simulink model "sfcndemo_sfun_udt"  (Simulink 6.0)
settings: Solver=ode1  StartTime=0.0  StopTime=10.0  FixedStep=0.05  RelTol=1e-3
settings Model: Creator=The MathWorks Inc.  LastModifiedBy=batserve  ExtModeAutoUpdateStatusClock=off
settings SolverCC: ZeroCrossControl=DisableAll
settings DataIOCC: SaveOutput=off  SaveTime=off
settings OptimizationCC: BlockReduction=off  BooleanDataType=off  InlineInvariantSignals=off
settings DebuggingCC: CheckExecutionContextPreStartOutputMsg=on  CheckExecutionContextRuntimeOutputMsg=on  SolverPrmCheckMsg=none
settings HardwareCC: TargetUnknown=on
settings RTWCC: RetainRTWFile=on

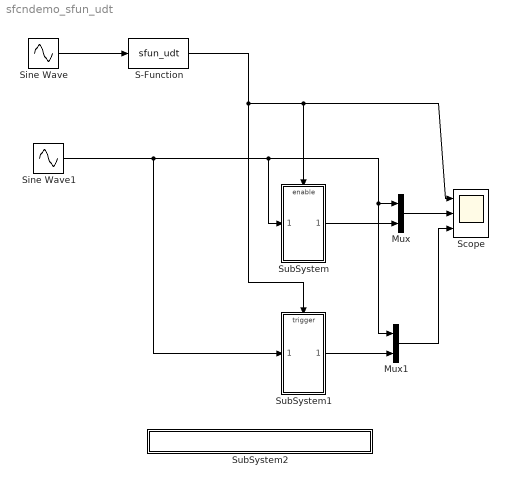
== system sfcndemo_sfun_udt ==
  Mux : Mux  Inputs=2
  Mux1 : Mux  Inputs=2
  S-Function : S-Function  FunctionName=sfun_udt
  Scope : Scope  NumInputPorts=3
      settings: YMin=-5~-5~-5  YMax=5~5~5
  Sine Wave : Sin  Amplitude=4.5  Frequency=1.5  SampleTime=0.05
  Sine Wave1 : Sin  Amplitude=4  SampleTime=0.05
  SubSystem : Subsystem  TreatAsAtomicUnit=on  PropExecContextAcrossSSBoundary=on
  SubSystem1 : Subsystem  TreatAsAtomicUnit=on  PropExecContextAcrossSSBoundary=on
  SubSystem2 : Subsystem  PropExecContextAcrossSSBoundary=on
      settings: OpenFcn=edit(fullfile(matlabroot,'simulink','src','sfun_udt.c'))
      mask Display: disp('matlabroot\simulink\src\sfun_udt.c');
  wires:
  Sine Wave/1 -> S-Function/1
  S-Function/1 -> SubSystem1/Trigger, SubSystem/Enable, Scope/1
  Sine Wave1/1 -> SubSystem1/1(In1), SubSystem/1(In1), Mux/1, Mux1/1
  Mux/1 -> Scope/2
  SubSystem/1(Out1) -> Mux/2
  SubSystem1/1(Out1) -> Mux1/2
  Mux1/1 -> Scope/3

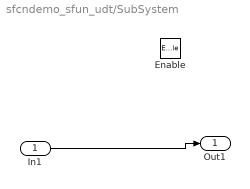
== system sfcndemo_sfun_udt/SubSystem ==
  In1 : Inport  Port=1  LatchInput=off
  Enable : EnablePort
  Out1 : Outport
  wires:
  In1/1 -> Out1/1

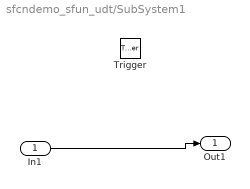
== system sfcndemo_sfun_udt/SubSystem1 ==
  In1 : Inport  Port=1  LatchInput=off
  Trigger : TriggerPort
  Out1 : Outport
  wires:
  In1/1 -> Out1/1

== system sfcndemo_sfun_udt/SubSystem2 ==
